simulink model "cps_blocks_v2"  (R2012b)
settings: Solver=FixedStepDiscrete  StartTime=0.0  StopTime=8.5  FixedStep=0.05  RelTol=20e-5
model workspace (MAT data in the model file):
  block = 1
libraries: visionstatistics x1, simulink x1
settings Model: Creator=pmosterm  LastModifiedBy=pmosterm
settings SolverCC: ZcThreshold=2e-5  MaxConsecutiveZCs=20  EnableConcurrentExecution=on  ConcurrentTasks=on  ZeroCrossAlgorithm=Adaptive  SolverResetMethod=Robust
settings OptimizationCC: InlineParams=on
settings DebuggingCC: AlgebraicLoopMsg=error  UnderspecifiedInitializationDetection=Simplified  FcnCallInpInsideContextMsg=EnableAllAsWarning  ModelReferenceExtraNoncontSigs=warning
settings GRTTargetCC: CombineOutputUpdateFcns=off  GRTInterface=on
settings ConfigurationSet: Description=SimMechanics 2G

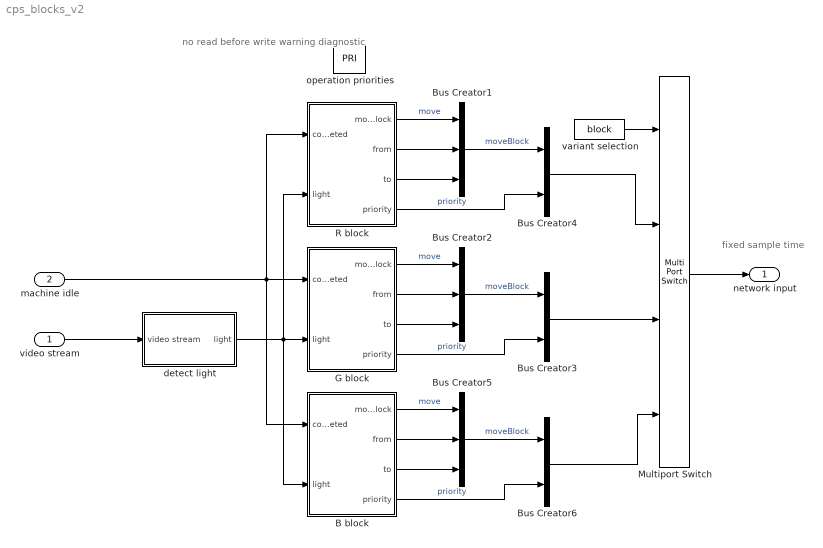
== system cps_blocks_v2 ==
  note: no read before write
      | warning diagnostic
  note: fixed sample time
  video stream : Inport  OutDataTypeStr=uint8  PortDimensions=[240 120 3]  SampleTime=0.1
  machine idle : Inport  Port=2
  B block : Stateflow chart  TreatAsAtomicUnit=on
  Bus Creator1 : BusCreator  Inputs='move','from','to'  OutDataTypeStr=Bus: slBusMoveBlock
  Bus Creator2 : BusCreator  Inputs='move','from','to'  OutDataTypeStr=Bus: slBusMoveBlock
  Bus Creator3 : BusCreator  Inputs=2  OutDataTypeStr=Bus: slBusBlockOps
  Bus Creator4 : BusCreator  Inputs=2  OutDataTypeStr=Bus: slBusBlockOps
  Bus Creator5 : BusCreator  Inputs='move','from','to'  OutDataTypeStr=Bus: slBusMoveBlock
  Bus Creator6 : BusCreator  Inputs=2  OutDataTypeStr=Bus: slBusBlockOps
  G block : Stateflow chart  TreatAsAtomicUnit=on
  Multiport Switch : MultiPortSwitch
  R block : Stateflow chart  TreatAsAtomicUnit=on
  detect light : Subsystem
  operation priorities : DataStoreMemory  DataStoreName=PRI  WriteAfterWriteMsg=warning  WriteAfterReadMsg=warning  InitialValue=[0 1 2 3 4]  OutDataTypeStr=int8
  variant selection : Constant  Value=block
  network input : Outport  OutDataTypeStr=Bus: slBusBlockOps  SampleTime=0.05  BusOutputAsStruct=on
  wires:
  G block/1(move_block) -> Bus Creator2/1  "move"
  G block/3(to) -> Bus Creator2/3
  G block/2(from) -> Bus Creator2/2
  R block/1(move_block) -> Bus Creator1/1  "move"
  R block/3(to) -> Bus Creator1/3
  R block/2(from) -> Bus Creator1/2
  machine idle/1 -> R block/1(completed), G block/1(completed), B block/1(completed)
  G block/4(priority) -> Bus Creator3/2  "priority"
  Bus Creator2/1 -> Bus Creator3/1  "moveBlock"
  R block/4(priority) -> Bus Creator4/2  "priority"
  Bus Creator1/1 -> Bus Creator4/1  "moveBlock"
  variant selection/1 -> Multiport Switch/1
  Multiport Switch/1 -> network input/1
  Bus Creator4/1 -> Multiport Switch/2
  B block/1(move_block) -> Bus Creator5/1  "move"
  B block/3(to) -> Bus Creator5/3
  B block/2(from) -> Bus Creator5/2
  B block/4(priority) -> Bus Creator6/2  "priority"
  Bus Creator5/1 -> Bus Creator6/1  "moveBlock"
  Bus Creator6/1 -> Multiport Switch/4
  Bus Creator3/1 -> Multiport Switch/3
  detect light/1(light) -> B block/2(light), R block/2(light), G block/2(light)
  video stream/1 -> detect light/1(video stream)

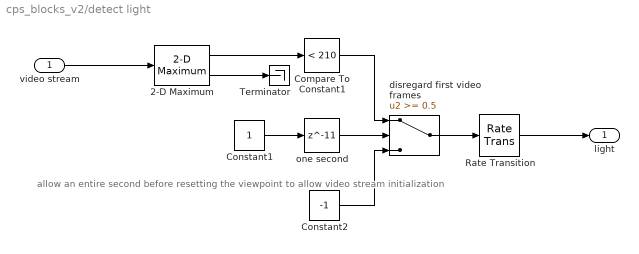
== system cps_blocks_v2/detect light ==
  note: allow an entire
      | second before
      | resetting the viewpoint
      | to allow video stream
      | initialization
  video stream : Inport
  2-D Maximum : visionstatistics/2-D Maximum  fcn=Value and Index  reset=None  indexBase=One  operateOver=Entire input  Dimension=1  colComp=on  operation=maximum  roiEnable=off  roiType=Rectangles  roiPortion=Entire ROI  roiOutput=Individual statistics for each ROI  roiFlag=off  accumDataTypeStr=Inherit: Same as product output  accumLastDataTypeStr=Inherit: Same as product output  roundingMode=Floor  overflowMode=off
  Compare To Constant1 : simulink/Logic and Bit Operations/Compare To Constant  relop=<  const=210  OutDataTypeStr=boolean
  Constant1 : Constant
  Constant2 : Constant  Value=-1
  Rate Transition : RateTransition  Deterministic=off
  Terminator : Terminator
  disregard first video frames : Switch  Threshold=0.5
  one second : Delay  DelayLength=11
  light : Outport
  wires:
  2-D Maximum/1 -> Compare To Constant1/1
  Compare To Constant1/1 -> disregard first video frames/1
  Constant2/1 -> disregard first video frames/3
  one second/1 -> disregard first video frames/2
  video stream/1 -> 2-D Maximum/1
  Constant1/1 -> one second/1
  2-D Maximum/2 -> Terminator/1
  disregard first video frames/1 -> Rate Transition/1
  Rate Transition/1 -> light/1

== stateflow chart cps_blocks_v2/B block ==
  state RequestDetermination [parallel]
    settings: executionOrder=1
    state Initial
      move_request = 0;
    state MoveLeftTwo
      move_request = 1;
    state Terminal
      move_request = 0;
    (default) -> Initial : /from = 0; to = 0;
        | priority = PRI[4];
    Initial -> (junction 3) [order 1]
    (junction 3) -> MoveLeftTwo : [light == 1]/
        | to = to - 2;
    Initial -> Initial [order 2] : [light == -1 || light == 0]
    MoveLeftTwo -> (junction 14) : [completed]/
        | from = from - 2;
    (junction 14) -> Terminal
  state RequestProcessing [parallel]
    settings: executionOrder=2
    state RequestSuspended
      move_block = 0;
    state RequestActive
      en: move_block = move_request;
      du: move_block = move_request;
    (default) -> RequestSuspended
    RequestSuspended -> RequestActive : [light == 1]
    RequestActive -> RequestSuspended : [light == 0]
  data: move_block output double; completed input; light input; from output double; to output double; PRI data_store_memory; priority output double; move_request local double

== stateflow chart cps_blocks_v2/G block ==
  state RequestDetermination [parallel]
    settings: executionOrder=1
    state Initial
      move_request = 0;
    state TwoStepPlan
    state MoveLeftOne
      move_request = 1;
    state Sync
    state MoveLeftOneMore
      move_request = 1;
    state Terminal
      move_request = 0;
    (default) -> Initial : /from = 0; to = 0;
        | priority = PRI[3];
    Initial -> (junction 3) [order 2]
    (junction 3) -> TwoStepPlan : [light == 1 || light ==0]
    Initial -> Initial [order 1] : [light == -1]
    TwoStepPlan -> MoveLeftOne : [light == 1]/
        | to = to -1;
    MoveLeftOne -> Sync : [completed]/
        | from = from - 1; to = to -1;
        | priority = PRI[1];
    Sync -> MoveLeftOneMore : [~completed]
    MoveLeftOneMore -> (junction 14) : [completed]/
        | from = from - 1;
    (junction 14) -> Terminal
  state RequestProcessing [parallel]
    settings: executionOrder=2
    state RequestSuspended
      move_block = 0;
    state RequestActive
      en: move_block = move_request;
      du: move_block = move_request;
    (default) -> RequestSuspended
    RequestSuspended -> RequestActive : [light == 1]
    RequestActive -> RequestSuspended : [light == 0]
  data: move_block output double; from output double; completed input; light input; to output double; PRI data_store_memory; priority output double; move_request local double

== stateflow chart cps_blocks_v2/R block ==
  state RequestDetermination [parallel]
    settings: executionOrder=1
    state Initial
      move_request = 0;
    state TwoStepPlan
    state ThreeStepPlan
    state MoveLeftOne
      move_request = 1;
    state MoveLeftOneAlt
      move_request = 1;
    note: The super makes
        | you wait 0.1 seconds
        | before going
        | back into your plan
    state TwoStepSync
    state ThreeStepSync1
    state MoveLeftOneMore
      move_request = 1;
    state MoveRightOne
      move_request = 1;
    state ThreeStepSync2
    state MoveLeftTwo
      move_request = 1;
    state Terminal
      move_request = 0;
    (default) -> Initial : /from = 0; to = 0;
        | priority = PRI[2];
    Initial -> (junction 3) [order 2]
    Initial -> (junction 10) [order 3]
    (junction 3) -> TwoStepPlan : [light == 1]
    (junction 10) -> ThreeStepPlan : [light == 0]
    Initial -> Initial [order 1] : [light == -1]
    TwoStepPlan -> MoveLeftOne : [light == 1]/
        | to = to -1;
    ThreeStepPlan -> MoveLeftOneAlt : [light == 1]/
        | to = to - 1;
    MoveLeftOne -> TwoStepSync : [completed]/
        | from = from - 1; to = to -1;
        | priority = PRI[1];
    MoveLeftOneAlt -> ThreeStepSync1 : [completed]/
        | from = from - 1; to = to +1;
        | priority = PRI[1];
    TwoStepSync -> MoveLeftOneMore : [~completed]
    ThreeStepSync1 -> MoveRightOne : [~completed]
    MoveLeftOneMore -> (junction 14) : [completed]/
        | from = from - 1;
    MoveRightOne -> ThreeStepSync2 : [completed]/
        | from = from + 1; to = to - 2;
        | priority = PRI[0];
    ThreeStepSync2 -> MoveLeftTwo : [~completed]
    MoveLeftTwo -> (junction 17) : [completed]/from = from - 2;
    (junction 14) -> Terminal
    (junction 17) -> Terminal
  state RequestProcessing [parallel]
    settings: executionOrder=2
    state RequestSuspended
      move_block = 0;
    state RequestActive
      en: move_block = move_request;
      du: move_block = move_request;
    (default) -> RequestSuspended
    RequestSuspended -> RequestActive : [light == 1]
    RequestActive -> RequestSuspended : [light == 0]
  data: move_block output double; from output double; completed input; light input; to output double; PRI data_store_memory; priority output double; move_request local double
